simulink model "m_testobj"  (Simulink 7.5)
settings: Solver=FixedStepDiscrete  StartTime=0.0  StopTime=10.0  RelTol=1e-3
undefined symbols (not defined in the file or in its folder): sldvsubsys
libraries: sldvlib x4
settings Model: Creator=yito  LastModifiedBy=itoy
settings OptimizationCC: InitFltsAndDblsToZero=on  OptimizeModelRefInitCode=on  LifeSpan=1
settings DebuggingCC: StrictBusMsg=Warning
settings RTWCC: SystemTargetFile=ert.tlc  TemplateMakefile=ert_default_tmf  Description=Real-Time Workshop Embedded Coder (no auto configuration)  ProcessScript=ert_make_rtw_hook
settings CodeAppCC: IgnoreCustomStorageClasses=off
settings ERTTargetCC: MultiwordLength=2048  GenerateSampleERTMain=on  InlinedParameterPlacement=NonHierarchical  ERTCustomFileTemplate=example_file_process.tlc  ConvertIfToSwitch=off
settings ConfigComp: Description=Design Verifier Custom Configuration Component  DVMaxProcessTime=600  DVDisplayUnsatisfiableObjectives=on  DVAutomaticStubbing=off  DVParameters=on  DVModelCoverageObjectives=None  DVMaxTestCaseSteps=500  DVTestSuiteOptimization=CombinedObjectives  DVSaveHarnessModel=on  DVSaveReport=on  DVActiveTab=3

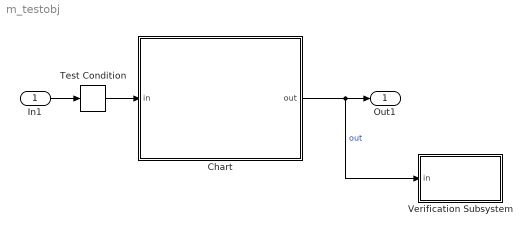
== system m_testobj ==
  In1 : Inport  DataType=uint8  OutDataType=sfix(16)  OutScaling=2^0  OutDataTypeStr=uint8
  Chart : Stateflow chart  TreatAsAtomicUnit=on
  Test Condition : sldvlib/Test Condition  SystemSampleTime=-1  enabled=on  customAVTBlockType=Test Condition  intervals={1,2,3}  initial=off  dispValues=on  outEnabled=on
      settings: AttributesFormatString=%<intervals>
  Verification Subsystem : Subsystem  Tag=VerificationSubsystem  DisableCoverage=on  LoadFcn=sldvsubsys('check')  TreatAsAtomicUnit=on  SimViewingDevice=on  mask(VerificationSubsystem){}
      mask init:
      | sldvsubsys('maskInit');
      settings: CopyFcn=sldvsubsys('copy');  OpenFcn=open_system(gcb,'force')
      settings: PreSaveFcn=|
      | set_param(gcb,'SimViewingDevice','on');
      | sldvsubsys('check');
      mask Help: helpview(fullfile(docroot,'toolbox','sldv','sldv.map'),'verificationsubsystem')
      mask Display: image(imread('sldvicon_versubsys.png','BackGroundColor',[1 1 1]),'center');
  Out1 : Outport  OutDataType=sfix(16)  OutScaling=2^0
  wires:
  Chart/1(out) -> Verification Subsystem/1(in), Out1/1  "out"
  In1/1 -> Test Condition/1
  Test Condition/1 -> Chart/1(in)

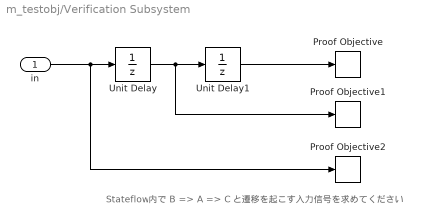
== system m_testobj/Verification Subsystem ==
  note: Stateflow内で B => A => C と遷移を起こす入力信号を求めてください
  in : Inport  OutDataType=sfix(16)  OutScaling=2^0
  Proof Objective : sldvlib/Proof Objective  SystemSampleTime=-1  enabled=on  customAVTBlockType=Test Objective  intervals=2  dispValues=on  outEnabled=off  enableStopSim=off
      settings: AttributesFormatString=%<intervals>
  Proof Objective1 : sldvlib/Proof Objective  SystemSampleTime=-1  enabled=on  customAVTBlockType=Test Objective  intervals=1  dispValues=on  outEnabled=off  enableStopSim=off
      settings: AttributesFormatString=%<intervals>
  Proof Objective2 : sldvlib/Proof Objective  SystemSampleTime=-1  enabled=on  customAVTBlockType=Test Objective  intervals=3  dispValues=on  outEnabled=off  enableStopSim=off
      settings: AttributesFormatString=%<intervals>
  Unit Delay : UnitDelay
  Unit Delay1 : UnitDelay
  wires:
  in/1 -> Unit Delay/1, Proof Objective2/1
  Unit Delay/1 -> Unit Delay1/1, Proof Objective1/1
  Unit Delay1/1 -> Proof Objective/1

== stateflow chart Chart ==
  state A/
    en: out=1;
  state B/
    en: out=2;
  state C/
    en: out=3;
  (default) -> A
  A -> C [order 2] : [in==3]
  C -> A : [in==1]
  A -> B [order 1] : [in==2]
  B -> A : [in==1]
  data: in input double; out output uint8
